simulink model "Model_ZN_PID"  (Simulink 9.2)
settings: Solver=VariableStepAuto  StartTime=0.0  StopTime=20  FixedStep=1e-3  MaxStep=1e-3  RelTol=1e-3  EnableMultiTasking=on
values from neighbouring files (symbols this model uses):
  disturb_step_time = handles.disTime    [GUI_Comparison1.m]    (also in GUI_Comparison2.m; GUI_Main.m = str2double(get(handles.edit_disTime,   'string')); function_PI_lambdaD.m = 100; programEx6PILamD.m = 40)
  disturb_step_value = handles.disValue    [GUI_Comparison1.m]    (also in GUI_Comparison2.m; GUI_Main.m = str2double(get(handles.edit_disValue,  'string')); function_PI_lambdaD.m = 0.5; programEx6PILamD.m = 0.5)
  L = handles.L    [GUI_Comparison1.m]    (also in GUI_Comparison2.m; GUI_Main.m; function_PI_lambdaD.m = delay; irid_fod.m = 200)
  step_value = handles.stepValue    [GUI_Comparison1.m]    (also in GUI_Comparison2.m; GUI_Main.m = str2double(get(handles.edit_stepValue, 'string')); programEx6PILamD.m = 1)
  ZN_kdo = ZN_Kp*ZN_Td    [GUI_Comparison2.m]
  ZN_kio = ZN_Kp/ZN_Ti    [GUI_Comparison2.m]
  ZN_kpo = ZN_Kp    [GUI_Comparison2.m]
libraries: cstblocks x1, simulink x1, powerlib x1
settings Model: Creator=Li Chuang  LastModifiedBy=18764
settings SolverCC: AlgebraicLoopSolver=LineSearch
settings OptimizationCC: InitFltsAndDblsToZero=on
settings DebuggingCC: SaveWithParameterizedLinksMsg=none  SignalResolutionControl=TryResolveAllWithWarning  SolverPrmCheckMsg=warning  MultiTaskDSMMsg=warning  MultiTaskCondExecSysMsg=none  FcnCallInpInsideContextMsg=error  AllowSymbolicDim=off  StateNameClashWarn=none
settings GRTTargetCC: TargetFcnLib=ansi_tfl_tmw.mat  GeneratePreprocessorConditionals=Use local settings

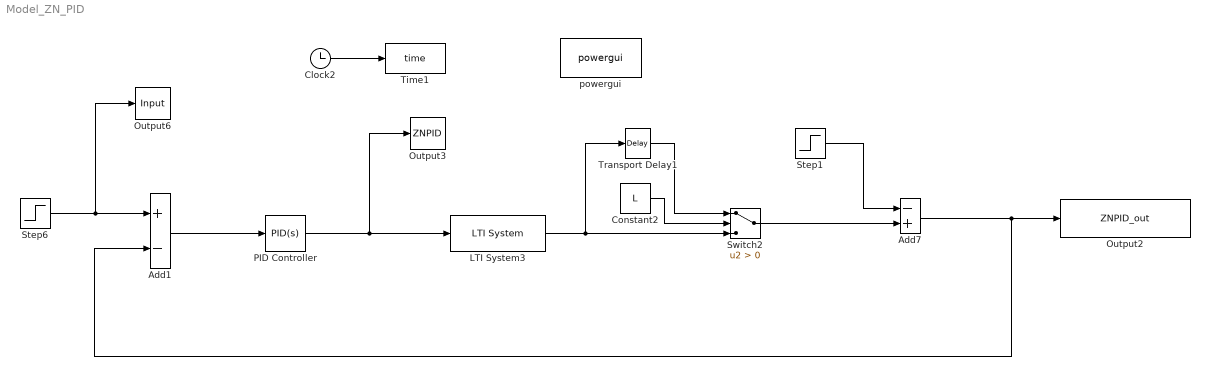
== system Model_ZN_PID ==
  Add1 : Sum  Inputs=+-  SaturateOnIntegerOverflow=on  OutDataTypeStr=Inherit: Same as first input
  Add7 : Sum  Inputs=-+  SaturateOnIntegerOverflow=on  OutDataTypeStr=Inherit: Same as first input
  Clock2 : Clock
      settings: Decimation=100
  Constant2 : Constant  Value=L
  LTI System3 : cstblocks/LTI System  sys=Gp  IC=[]
  Output2 : ToWorkspace  VariableName=ZNPID_out  SampleTime=-1
  Output3 : ToWorkspace  VariableName=ZNPID  SampleTime=-1
  Output6 : ToWorkspace  VariableName=Input  SampleTime=-1
  PID Controller : simulink/Continuous/PID Controller  Controller=PID  Form=Parallel  TimeDomain=Continuous-time  SampleTime=-1  IntegratorMethod=Forward Euler  FilterMethod=Forward Euler  ControllerParametersSource=internal  P=ZN_kpo  I=ZN_kio  D=ZN_kdo  UseFilter=on  N=100  TunerSelectOption=Transfer Function Based (PID Tuner App)  InitialConditionSource=internal  InitialConditionForIntegrator=0  InitialConditionForFilter=0  DifferentiatorICPrevScaledInput=0  ExternalReset=none  TrackingMode=off  Kt=1  LimitOutput=off  UpperSaturationLimit=inf  LowerSaturationLimit=-inf  LinearizeAsGain=on  AntiWindupMode=none  Kb=1  POutMin=[]  POutMax=[]  IOutMin=[]  IOutMax=[]  DOutMin=[]  DOutMax=[]  NOutMin=[]  NOutMax=[]  SumOutMin=[]  SumOutMax=[]  SaturationOutMin=[]  SaturationOutMax=[]  PParamMin=[]  PParamMax=[]  IParamMin=[]  IParamMax=[]  DParamMin=[]  DParamMax=[]  NParamMin=[]  NParamMax=[]  KbParamMin=[]  KbParamMax=[]  KtParamMin=[]  KtParamMax=[]  KbOutMin=[]  KbOutMax=[]  KtOutMin=[]  KtOutMax=[]  IntegratorOutMin=[]  IntegratorOutMax=[]  FilterOutMin=[]  FilterOutMax=[]  SumI1OutMin=[]  SumI1OutMax=[]  SumI2OutMin=[]  SumI2OutMax=[]  SumI3OutMin=[]  SumI3OutMax=[]  SumI4OutMin=[]  SumI4OutMax=[]  SumDOutMin=[]  SumDOutMax=[]  DifferentiatorOutMin=[]  DifferentiatorOutMax=[]  FilterDiffOutCoefMin=[]  FilterDiffOutCoefMax=[]  ReciprocalOutMin=[]  ReciprocalOutMax=[]  SumDenOutMin=[]  SumDenOutMax=[]  SumNumOutMin=[]  SumNumOutMax=[]  DivideOutMin=[]  DivideOutMax=[]  IntegratorContinuousStateAttributes=''  IntegratorStateMustResolveToSignalObject=off  IntegratorRTWStateStorageClass=Auto  FilterContinuousStateAttributes=''  FilterStateMustResolveToSignalObject=off  FilterRTWStateStorageClass=Auto  ParallelPVariant=InternalParameters  IdealPVariant=Disabled  IVariant=InternalParameters  DVariant=InternalParameters  IntegratorVariant=Continuous  SatVariant=Disabled  AWVariant=Passthrough  PCopyVariant=Disabled  TRVariant=Disabled  FdbkBlocksVariant=Forward  IdealPFdbkVariant=Disabled  SatFdbkVariant=Disabled  DerivativeFilterVariant=ContFilter  NVariant=InternalParameters  NCopyVariant=Disabled  FilterICVariant=InternalICsFilter  IntegratorICVariant=InternalICs  ExternalResetVariant=Disabled  TRSumVariant=Passthrough  SumFdbkVariant=Disabled  SumVariant=Sum_PID
  Step1 : Step  Time=disturb_step_time  After=disturb_step_value
  Step6 : Step  Time=0  After=step_value
  Switch2 : Switch  Criteria=u2 > Threshold
  Time1 : ToWorkspace  VariableName=time  SampleTime=-1
  Transport Delay1 : TransportDelay  DelayTime=L
  powergui : powerlib/powergui  Priority=1  SimulationMode=Discrete  SampleTime=50e-6  frequency=60  Iterations=50  frequencyindice=60  Pbase=100e6  ErrMax=1e-4  UnitsV=kV  UnitsW=MW  buscounter=0  FunctionMessages=off  echomessages=off  EnableUseOfTLC=off  CurrentSourceSwitches=off  DisableSnubberDevices=off  DisableRonSwitches=off  DisableVfSwitches=off  DisplayEquations=off  SolverType=Tustin/Backward Euler (TBE)  Interpol=off  ExternalGateDelay=off  methode=off  Ts=100  x0status=blocks  SPID=off  SwTol=0  HookPort=off  RestoreLinks=warning  ResistiveCurrentMeasurement=off  Frange=[0:2:500]  Ylog=off  Xlog=on  ShowGrid=off  save=off  variable=ZData  structure=0  ZoomFFT=off  StartTime=0.0  cycles=1  DisplayStyle=1  fundamental=60  FreqAxis=off  MaxFrequency=1000  frequencyindicesteady=1  RmsSteady=1  display=off
  wires:
  Clock2/1 -> Time1/1
  Step6/1 -> Output6/1, Add1/1
  PID Controller/1 -> LTI System3/1, Output3/1
  Transport Delay1/1 -> Switch2/1
  Add1/1 -> PID Controller/1
  Add7/1 -> Add1/2, Output2/1
  Constant2/1 -> Switch2/2
  Switch2/1 -> Add7/2
  LTI System3/1 -> Switch2/3, Transport Delay1/1
  Step1/1 -> Add7/1
